simulink model "sixrooms_dynamics"  (R2023a)
settings: Solver=VariableStepAuto  StartTime=0.0  StopTime=10.0  RelTol=1e-3
libraries: simulink x2
settings Model: Creator=oluwafemiajeigbe  LastModifiedBy=oluwafemiajeigbe

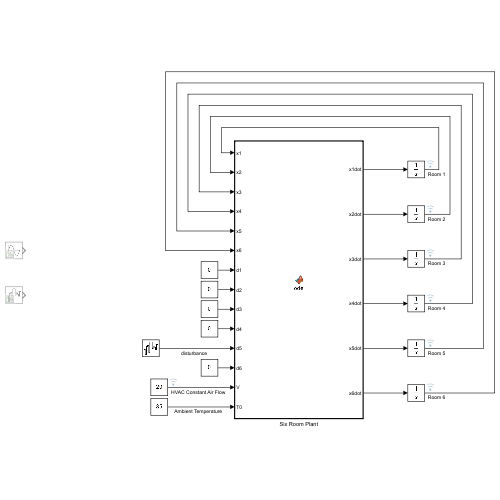
[thumbnail: Simulink's stored preview of the top-level diagram]
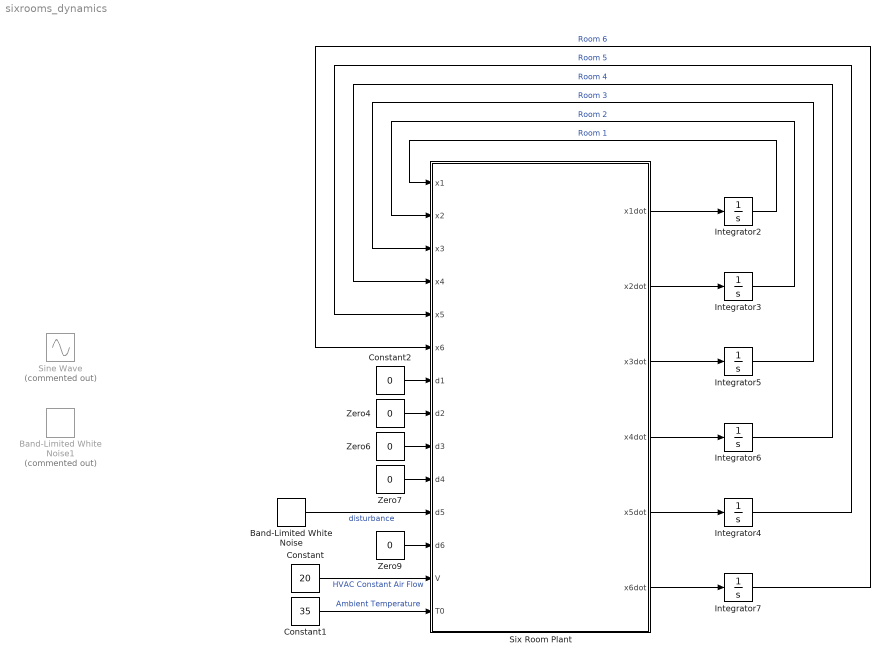
== system sixrooms_dynamics ==
  Band-Limited White Noise : simulink/Sources/Band-Limited White Noise  Cov=[0.7]  Ts=0.1  seed=[23341]
  Band-Limited White Noise1 : simulink/Sources/Band-Limited White Noise  Commented=on  Cov=[18]  Ts=0.1  seed=[23341]
  Constant : Constant  Value=20
  Constant1 : Constant  Value=35
  Constant2 : Constant  Value=0
  Integrator{2..7} (6 alike) : Integrator
  Sine Wave : Sin  Commented=on  Amplitude=(42-35)/2  Bias=35+ (42-35)/2  Phase=24  SampleTime=0
  Six Room Plant : MATLAB Function  TreatAsAtomicUnit=on
  Zero{4,6..7,9} (4 alike) : Constant  Value=0  OutDataTypeStr=Inherit: Inherit via back propagation
  wires:
  Constant1/1 -> Six Room Plant/14(T0)  "Ambient Temperature"
  Band-Limited White Noise/1 -> Six Room Plant/11(d5)  "disturbance"
  Zero4/1 -> Six Room Plant/8(d2)
  Integrator7/1 -> Six Room Plant/6(x6)  "Room 6"
  Integrator2/1 -> Six Room Plant/1(x1)  "Room 1"
  Constant/1 -> Six Room Plant/13(V)  "HVAC Constant Air Flow"
  Zero7/1 -> Six Room Plant/10(d4)
  Six Room Plant/4(x4dot) -> Integrator6/1
  Zero9/1 -> Six Room Plant/12(d6)
  Integrator6/1 -> Six Room Plant/4(x4)  "Room 4"
  Six Room Plant/3(x3dot) -> Integrator5/1
  Integrator5/1 -> Six Room Plant/3(x3)  "Room 3"
  Integrator3/1 -> Six Room Plant/2(x2)  "Room 2"
  Six Room Plant/6(x6dot) -> Integrator7/1
  Zero6/1 -> Six Room Plant/9(d3)
  Six Room Plant/1(x1dot) -> Integrator2/1
  Six Room Plant/2(x2dot) -> Integrator3/1
  Six Room Plant/5(x5dot) -> Integrator4/1
  Constant2/1 -> Six Room Plant/7(d1)
  Integrator4/1 -> Six Room Plant/5(x5)  "Room 5"

== matlab function sixrooms_dynamics/Six Room Plant ==
  data: x1 input; x1dot output; x2 input; x3 input; x4 input; x5 input; x6 input; d1 input; d2 input; d3 input; d4 input; d5 input; d6 input; x2dot output; V input; x3dot output; x4dot output; x5dot output; x6dot output; T0 input
function [x1dot, x2dot, x3dot, x4dot, x5dot, x6dot] = ode(x1, x2, x3, x4, x5, x6, d1, d2,  d3,  d4, d5, d6, V, T0)

% Define Parameters
m = 100; % Thermal capacitance of room i
w12 = 0.9; % Thermal conductance between room 1 and room 2
w14 = 1.7; % Thermal conductance between room 1 and room 4
w21 = 0.9; % Thermal conductance between room 2 and room 1
w23 = 0.4; % Thermal conductance between room 2 and room 3
w25 = 1.9; % Thermal conductance between room 2 and room 5
w32 = 0.4; % Thermal conductance between room 3 and room 2
w36 = 1.4; % Thermal conductance between room 3 and room 6
w45 = 1.5; % Thermal conductance between room 4 and room 5
w54 = 1.5; % Thermal conductance between room 5 and room 4
w56 = 1.6; % Thermal conductance between room 5 and room 6
w63 = 1.4; % Thermal conductance between room 6 and room 3
w41 = 1.7; % Thermal conductance between room 6 and room 3
w52 = 1.9; % Thermal conductance between room 6 and room 3
w65 = 1.6; % Thermal conductance between room 6 and room 5

rho = 1.2; % air density
cp = 10;  % specific heat capacity of air

wio = 0.05; % Thermal conductance between room i and outside

gamma1 = 0.5; %fraction of the HVAC air volume to room 1
gamma2 = 0.5; %fraction of the HVAC air volume to room 2
gamma3 = 0.5; %fraction of the HVAC air volume to room 3
gamma4 = 0.5; %fraction of the HVAC air volume to room 4
gamma5 = 0.5; %fraction of the HVAC air volume to room 5
gamma6 = 0.5; %fraction of the HVAC air volume to room 6

%T0 = 22; % Constant temperature of the HVAC air flow


% u=V is the control input

x1dot = 1/m*(w21*(x2-x1) + w41*(x4-x1) - wio*x1 + gamma1*rho*V*cp*(T0-x1)+d1);
x2dot = 1/m*(w12*(x1-x2) +w32*(x3-x2) +w52*(x5-x2) - wio*x2 + gamma2*rho*V*cp*(T0-x2)+d2);
x3dot = 1/m*(w23*(x2-x3) + w63*(x6-x3) - wio*x3 + gamma3*rho*V*cp*(T0-x3)+d3);
x4dot = 1/m*(w14*(x1-x4) + w54*(x5-x4) - wio*x4 + gamma4*rho*V*cp*(T0-x4)+d4);
x5dot = 1/m*(w25*(x2-x5) + w45*(x4-x5) + w65*(x6-x5) - wio*x5 + gamma5*rho*V*cp*(T0-x5)+d5);
x6dot = 1/m*(w36*(x3-x6) + w56*(x5-x6) - wio*x6 + gamma6*rho*V*cp*(T0-x6)+d6);
